simulink model "controller_dev_sg"  (R2018b)
settings: configuration reference "Physics" (kept outside this file)
model workspace (MAT data in the model file):
  m = 1000
undefined symbols (not defined in the file or in its folder): C, P_MLOC_NumberOfNoSendFrames, tS, TUMHealthStatus, TUMStateEstimationState, TUMVehicleState, x0_vehiclepose_stm
libraries: xpcrtudplib x13, simulink x12, canmsglib x12, etargetslib x10, speedgoatlib_IO614 x9, misc x4, xpcutilitieslib x1
(part 2 of 2)

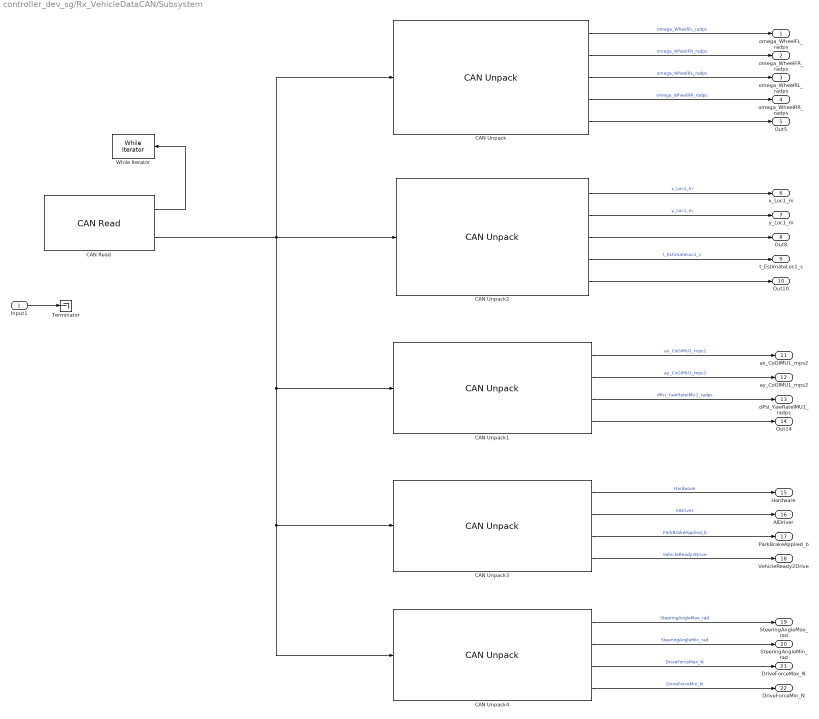
== system controller_dev_sg/Rx_VehicleDataCAN/Subsystem ==
  Input1 : Inport
  CAN Read : speedgoatlib_IO614/CAN/CAN Read  id=1  sampleTime=-1  portSelection=4  messageType=CAN  protl=IO614  ptIdx=3  isFDMod=0
      settings: SourceProductName=Simulink Real-Time: Speedgoat Library
  CAN Unpack : canmsglib/CAN Unpack  MsgList=(none)  MsgName=CAN Msg  MsgIDType=Standard (11-bit identifier)  MsgIdentifier=768  MsgLength=8  SignalInfo=omega_WheelFL_radps$0$15$1$1$1$0$0.1$0$-Inf$Inf$#omega_WheelFR_radps$15$15$1$1$1$0$0.1$0$-Inf$Inf$#omega_WheelRL_radps$30$15$1$1$1$0$0.1$0$-Inf$Inf$#omega_WheelRR_radps$45$15$1$1$1$0$0.1$0$-Inf$Inf$#valid_Wheelspeeds_b$60$4$1$1$1$0$1$0$-Inf$Inf$#  NSignals=5  IDPort=off  TimestampPort=off  ErrorPort=off  RemotePort=off  LengthPort=off  StatusPort=off  StartBits=str2num('[int32(0);int32(15);int32(30);int32(45);int32(60)]')  SignalSizes=str2num('[int32(15);int32(15);int32(15);int32(15);int32(4)]')  ByteOrders=str2num('[int32(1);int32(1);int32(1);int32(1);int32(1)]')  DataTypes=str2num('[int32(1);int32(1);int32(1);int32(1);int32(1)]')  MultiplexTypes=str2num('[int32(1);int32(1);int32(1);int32(1);int32(1)]')  MultiplexValues=str2num('[double(0);double(0);double(0);double(0);double(0)]')  Factors=str2num('[double(0.1);double(0.1);double(0.1);double(0.1);double(1)]')  Offsets=str2num('[double(0);double(0);double(0);double(0);double(0)]')  Minimums=str2num('[double(-Inf);double(-Inf);double(-Inf);double(-Inf);double(-Inf)]')  Maximums=str2num('[double(Inf);double(Inf);double(Inf);double(Inf);double(Inf)]')  ApplyMinMax=off
      settings: SourceProductName=Simulink Real-Time
  CAN Unpack1 : canmsglib/CAN Unpack  MsgList=(none)  MsgName=CAN Msg  MsgIDType=Standard (11-bit identifier)  MsgIdentifier=48  MsgLength=8  SignalInfo=ax_CoGIMU1_mps2$0$16$1$1$1$0$0.001$0$-Inf$Inf$#ay_CoGIMU1_mps2$16$16$1$1$1$0$0.001$0$-Inf$Inf$#dPsi_YawRateIMU1_radps$32$16$1$1$1$0$0.0001$0$-Inf$Inf$#valid_IMU1_b$48$16$1$1$1$0$1$0$-Inf$Inf$#  NSignals=4  IDPort=off  TimestampPort=off  ErrorPort=off  RemotePort=off  LengthPort=off  StatusPort=off  StartBits=str2num('[int32(0);int32(16);int32(32);int32(48)]')  SignalSizes=str2num('[int32(16);int32(16);int32(16);int32(16)]')  ByteOrders=str2num('[int32(1);int32(1);int32(1);int32(1)]')  DataTypes=str2num('[int32(1);int32(1);int32(1);int32(1)]')  MultiplexTypes=str2num('[int32(1);int32(1);int32(1);int32(1)]')  MultiplexValues=str2num('[double(0);double(0);double(0);double(0)]')  Factors=str2num('[double(0.001);double(0.001);double(0.0001);double(1)]')  Offsets=str2num('[double(0);double(0);double(0);double(0)]')  Minimums=str2num('[double(-Inf);double(-Inf);double(-Inf);double(-Inf)]')  Maximums=str2num('[double(Inf);double(Inf);double(Inf);double(Inf)]')  ApplyMinMax=off
      settings: SourceProductName=Simulink Real-Time
  CAN Unpack2 : canmsglib/CAN Unpack  MsgList=(none)  MsgName=CAN Msg  MsgIDType=Standard (11-bit identifier)  MsgIdentifier=192  MsgLength=8  SignalInfo=x_Loc1_m$0$15$1$1$1$0$0.05$0$-Inf$Inf$#y_Loc1_m$15$15$1$1$1$0$0.05$0$-Inf$Inf$#psi_YawAngleLoc1_rad$30$15$1$1$1$0$0.001$0$-Inf$Inf$#t_EstimateLoc1_s$45$15$1$1$1$0$0.001$0$-Inf$Inf$#valid_Loc1_b$60$4$1$1$1$0$1$0$-Inf$Inf$#  NSignals=5  IDPort=off  TimestampPort=off  ErrorPort=off  RemotePort=off  LengthPort=off  StatusPort=off  StartBits=str2num('[int32(0);int32(15);int32(30);int32(45);int32(60)]')  SignalSizes=str2num('[int32(15);int32(15);int32(15);int32(15);int32(4)]')  ByteOrders=str2num('[int32(1);int32(1);int32(1);int32(1);int32(1)]')  DataTypes=str2num('[int32(1);int32(1);int32(1);int32(1);int32(1)]')  MultiplexTypes=str2num('[int32(1);int32(1);int32(1);int32(1);int32(1)]')  MultiplexValues=str2num('[double(0);double(0);double(0);double(0);double(0)]')  Factors=str2num('[double(0.05);double(0.05);double(0.001);double(0.001);double(1)]')  Offsets=str2num('[double(0);double(0);double(0);double(0);double(0)]')  Minimums=str2num('[double(-Inf);double(-Inf);double(-Inf);double(-Inf);double(-Inf)]')  Maximums=str2num('[double(Inf);double(Inf);double(Inf);double(Inf);double(Inf)]')  ApplyMinMax=off
      settings: SourceProductName=Simulink Real-Time
  CAN Unpack3 : canmsglib/CAN Unpack  MsgList=(none)  MsgName=CAN Msg  MsgIDType=Standard (11-bit identifier)  MsgIdentifier=12  MsgLength=8  SignalInfo=Hardware$0$12$1$2$1$0$1$0$-Inf$Inf$#AIDriver$12$12$1$2$1$0$1$0$-Inf$Inf$#ParkBrakeApplied_b$24$12$1$1$1$0$1$0$-Inf$Inf$#VehicleReady2Drive$36$12$1$1$1$0$1$0$-Inf$Inf$#  NSignals=4  IDPort=off  TimestampPort=off  ErrorPort=off  RemotePort=off  LengthPort=off  StatusPort=off  StartBits=str2num('[int32(0);int32(12);int32(24);int32(36)]')  SignalSizes=str2num('[int32(12);int32(12);int32(12);int32(12)]')  ByteOrders=str2num('[int32(1);int32(1);int32(1);int32(1)]')  DataTypes=str2num('[int32(2);int32(2);int32(1);int32(1)]')  MultiplexTypes=str2num('[int32(1);int32(1);int32(1);int32(1)]')  MultiplexValues=str2num('[double(0);double(0);double(0);double(0)]')  Factors=str2num('[double(1);double(1);double(1);double(1)]')  Offsets=str2num('[double(0);double(0);double(0);double(0)]')  Minimums=str2num('[double(-Inf);double(-Inf);double(-Inf);double(-Inf)]')  Maximums=str2num('[double(Inf);double(Inf);double(Inf);double(Inf)]')  ApplyMinMax=off
      settings: SourceProductName=Simulink Real-Time
  CAN Unpack4 : canmsglib/CAN Unpack  MsgList=(none)  MsgName=CAN Msg  MsgIDType=Standard (11-bit identifier)  MsgIdentifier=170  MsgLength=8  SignalInfo=SteeringAngleMax_rad$0$16$1$1$1$0$0.001$0$-Inf$Inf$#SteeringAngleMin_rad$16$16$1$1$1$0$0.001$0$-Inf$Inf$#DriveForceMax_N$32$16$1$1$1$0$100$0$-Inf$Inf$#DriveForceMin_N$48$16$1$1$1$0$100$0$-Inf$Inf$#  NSignals=4  IDPort=off  TimestampPort=off  ErrorPort=off  RemotePort=off  LengthPort=off  StatusPort=off  StartBits=str2num('[int32(0);int32(16);int32(32);int32(48)]')  SignalSizes=str2num('[int32(16);int32(16);int32(16);int32(16)]')  ByteOrders=str2num('[int32(1);int32(1);int32(1);int32(1)]')  DataTypes=str2num('[int32(1);int32(1);int32(1);int32(1)]')  MultiplexTypes=str2num('[int32(1);int32(1);int32(1);int32(1)]')  MultiplexValues=str2num('[double(0);double(0);double(0);double(0)]')  Factors=str2num('[double(0.001);double(0.001);double(100);double(100)]')  Offsets=str2num('[double(0);double(0);double(0);double(0)]')  Minimums=str2num('[double(-Inf);double(-Inf);double(-Inf);double(-Inf)]')  Maximums=str2num('[double(Inf);double(Inf);double(Inf);double(Inf)]')  ApplyMinMax=off
      settings: SourceProductName=Simulink Real-Time
  Terminator : Terminator
  While Iterator : WhileIterator  MaxIters=501  WhileBlockType=do-while
  omega_WheelFL_radps : Outport
  omega_WheelFR_radps : Outport  Port=2
  omega_WheelRL_radps : Outport  Port=3
  omega_WheelRR_radps : Outport  Port=4
  Out5 : Outport  Port=5
  x_Loc1_m : Outport  Port=6
  y_Loc1_m : Outport  Port=7
  Out8 : Outport  Port=8
  t_EstimateLoc1_s : Outport  Port=9
  Out10 : Outport  Port=10
  ax_CoGIMU1_mps2 : Outport  Port=11
  ay_CoGIMU1_mps2 : Outport  Port=12
  dPsi_YawRateIMU1_radps : Outport  Port=13
  Out14 : Outport  Port=14
  Hardware : Outport  Port=15
  AIDriver : Outport  Port=16
  ParkBrakeApplied_b : Outport  Port=17
  VehicleReady2Drive : Outport  Port=18
  SteeringAngleMax_rad : Outport  Port=19
  SteeringAngleMin_rad : Outport  Port=20
  DriveForceMax_N : Outport  Port=21
  DriveForceMin_N : Outport  Port=22
  wires:
  CAN Read/2 -> CAN Unpack/1, CAN Unpack2/1, CAN Unpack1/1, CAN Unpack3/1, CAN Unpack4/1
  CAN Unpack/4 -> omega_WheelRR_radps/1  "omega_WheelRR_radps"
  CAN Unpack2/2 -> y_Loc1_m/1  "y_Loc1_m"
  CAN Unpack2/5 -> Out10/1
  Input1/1 -> Terminator/1
  CAN Unpack/5 -> Out5/1
  CAN Read/1 -> While Iterator/1
  CAN Unpack1/1 -> ax_CoGIMU1_mps2/1  "ax_CoGIMU1_mps2"
  CAN Unpack2/4 -> t_EstimateLoc1_s/1  "t_EstimateLoc1_s"
  CAN Unpack2/3 -> Out8/1
  CAN Unpack/1 -> omega_WheelFL_radps/1  "omega_WheelFL_radps"
  CAN Unpack4/3 -> DriveForceMax_N/1  "DriveForceMax_N"
  CAN Unpack/3 -> omega_WheelRL_radps/1  "omega_WheelRL_radps"
  CAN Unpack1/2 -> ay_CoGIMU1_mps2/1  "ay_CoGIMU1_mps2"
  CAN Unpack4/2 -> SteeringAngleMin_rad/1  "SteeringAngleMin_rad"
  CAN Unpack3/2 -> AIDriver/1  "AIDriver"
  CAN Unpack3/3 -> ParkBrakeApplied_b/1  "ParkBrakeApplied_b"
  CAN Unpack1/4 -> Out14/1
  CAN Unpack4/1 -> SteeringAngleMax_rad/1  "SteeringAngleMax_rad"
  CAN Unpack/2 -> omega_WheelFR_radps/1  "omega_WheelFR_radps"
  CAN Unpack2/1 -> x_Loc1_m/1  "x_Loc1_m"
  CAN Unpack3/4 -> VehicleReady2Drive/1  "VehicleReady2Drive"
  CAN Unpack3/1 -> Hardware/1  "Hardware"
  CAN Unpack1/3 -> dPsi_YawRateIMU1_radps/1  "dPsi_YawRateIMU1_radps"
  CAN Unpack4/4 -> DriveForceMin_N/1  "DriveForceMin_N"

== system controller_dev_sg/Tx_TPCommsControllerSide/BehaviorStatemachine ==
  TrajPlannerSend : Inport
  DebugData : Inport  Port=2  OutDataTypeStr=Bus: mvdc_vehicle_dynamics_control_debug  PortDimensions=1
  Bus Selector1 : BusSelector  OutputSignals=TUMVehicleState
  Bus Selector2 : BusSelector  OutputSignals=ErrorCode
  Byte Pack : etargetslib/Byte Pack  datatypes={'uint16', 'uint32', 'uint16'}  byteAlign=1
  Constant : Constant  Value=boolean(1)  SampleTime=-1
  Counter Free-Running : simulink/Sources/Counter Free-Running  NumBits=8  tsamp=-1
  Data Type Conversion : DataTypeConversion  OutDataTypeStr=uint16
  Data Type Conversion1 : DataTypeConversion  OutDataTypeStr=uint32
  Data Type Conversion2 : DataTypeConversion  OutDataTypeStr=uint16
  BSM_ActivateSend : Outport
  BSM_Package : Outport  Port=2
  wires:
  Counter Free-Running/1 -> Data Type Conversion2/1
  Data Type Conversion/1 -> Byte Pack/1
  Data Type Conversion2/1 -> Byte Pack/3
  Byte Pack/1 -> BSM_Package/1
  Constant/1 -> BSM_ActivateSend/1
  TrajPlannerSend/1 -> Bus Selector1/1
  Bus Selector1/1 -> Data Type Conversion/1  "<TUMVehicleState>"
  DebugData/1 -> Bus Selector2/1
  Bus Selector2/1 -> Data Type Conversion1/1  "<ErrorCode>"
  Data Type Conversion1/1 -> Byte Pack/2

== system controller_dev_sg/Tx_TPCommsControllerSide/SendToBehaviorStatemachine1 ==
  Data : Inport
  Enable : EnablePort
  "Send " : xpcrtudplib/UDP Send  ipAddressVal=10.0.1.0  localPort=-1  toAddress=255.255.255.255  toPort=BehaviorStatemachineSend_Port  sampleTime=-1
      settings: SourceProductName=Simulink Real-Time  SourceProductBaseCode=XP
  Width : Width
  wires:
  Width/1 -> "Send "/2
  Data/1 -> Width/1, "Send "/1

== system controller_dev_sg/Tx_TPCommsControllerSide/SendToTrajectoryGeneration1 ==
  Data : Inport
  Enable : EnablePort
  "Send " : xpcrtudplib/UDP Send  ipAddressVal=10.0.1.0  localPort=-1  toAddress=255.255.255.255  toPort=TrajectoryGenerationSend_Port  sampleTime=-1
      settings: SourceProductName=Simulink Real-Time  SourceProductBaseCode=XP
  Width : Width
  wires:
  Width/1 -> "Send "/2
  Data/1 -> Width/1, "Send "/1

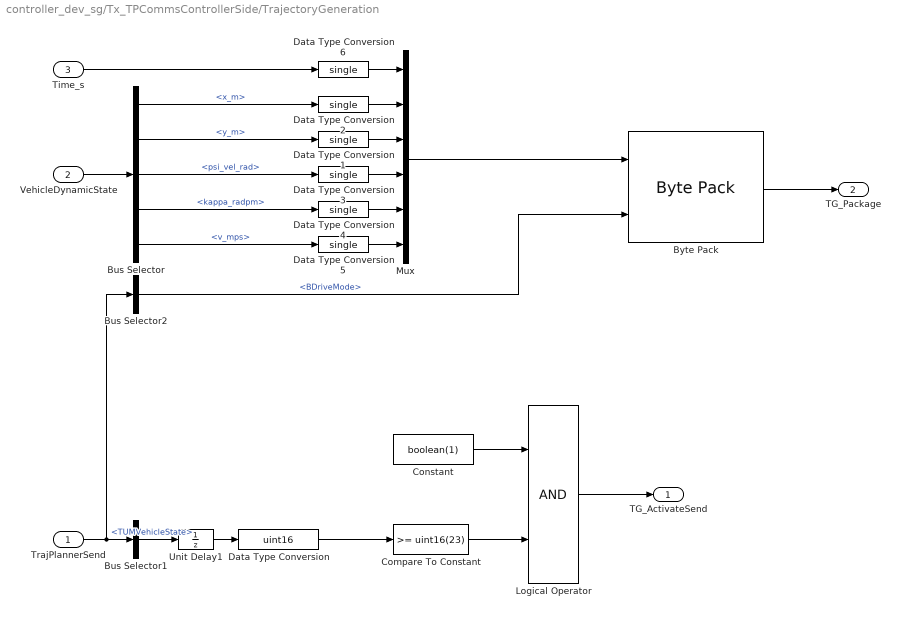
== system controller_dev_sg/Tx_TPCommsControllerSide/TrajectoryGeneration ==
  TrajPlannerSend : Inport
  VehicleDynamicState : Inport  Port=2
  Time_s : Inport  Port=3
  Bus Selector : BusSelector  OutputSignals=Pos.x_m,Pos.y_m,psi_vel_rad,kappa_radpm,v_mps
  Bus Selector1 : BusSelector  OutputSignals=TUMVehicleState
  Bus Selector2 : BusSelector  OutputSignals=BDriveMode
  Byte Pack : etargetslib/Byte Pack  datatypes={['single'], 'uint8'}  byteAlign=1
  Compare To Constant : simulink/Logic and Bit Operations/Compare To Constant  relop=>=  const=uint16(23)  OutDataTypeStr=boolean
  Constant : Constant  Value=boolean(1)  SampleTime=-1
  Data Type Conversion : DataTypeConversion  OutDataTypeStr=uint16
  Data Type Conversion{1..6} (6 alike) : DataTypeConversion  OutDataTypeStr=single
  Logical Operator : Logic  AllPortsSameDT=off  OutDataTypeStr=boolean
  Mux : Mux  Inputs=6
  Unit Delay1 : UnitDelay  InitialCondition=TUMVehicleState.OFF  SampleTime=tS
  TG_ActivateSend : Outport
  TG_Package : Outport  Port=2
  wires:
  Unit Delay1/1 -> Data Type Conversion/1
  Data Type Conversion/1 -> Compare To Constant/1
  Bus Selector/5 -> Data Type Conversion5/1  "<v_mps>"
  Data Type Conversion6/1 -> Mux/1
  Data Type Conversion4/1 -> Mux/5
  Data Type Conversion5/1 -> Mux/6
  Data Type Conversion1/1 -> Mux/3
  Data Type Conversion2/1 -> Mux/2
  Data Type Conversion3/1 -> Mux/4
  Time_s/1 -> Data Type Conversion6/1
  VehicleDynamicState/1 -> Bus Selector/1
  Mux/1 -> Byte Pack/1
  Bus Selector/4 -> Data Type Conversion4/1  "<kappa_radpm>"
  Byte Pack/1 -> TG_Package/1
  Bus Selector/1 -> Data Type Conversion2/1  "<x_m>"
  Bus Selector/2 -> Data Type Conversion1/1  "<y_m>"
  Bus Selector/3 -> Data Type Conversion3/1  "<psi_vel_rad>"
  Compare To Constant/1 -> Logical Operator/2
  Logical Operator/1 -> TG_ActivateSend/1
  Constant/1 -> Logical Operator/1
  TrajPlannerSend/1 -> Bus Selector2/1, Bus Selector1/1
  Bus Selector1/1 -> Unit Delay1/1  "<TUMVehicleState>"
  Bus Selector2/1 -> Byte Pack/2  "<BDriveMode>"

== system controller_dev_sg/Tx_TPCommsTPSide/BSM_Package ==
  TrajPlannerSend : Inport
  Bus Selector : BusSelector  OutputSignals=Strategy_Status
  Byte Pack : etargetslib/Byte Pack  datatypes={'uint16', 'uint16', 'uint32'}  byteAlign=1
  Constant : Constant  Value=0  SampleTime=-1
  Counter Free-Running : simulink/Sources/Counter Free-Running  NumBits=8  tsamp=-1
  Data Type Conversion : DataTypeConversion  OutDataTypeStr=uint16
  Data Type Conversion1 : DataTypeConversion  OutDataTypeStr=uint32
  Data Type Conversion2 : DataTypeConversion  OutDataTypeStr=uint16
  ResettableCounter : Subsystem
  BSM_ActivateSend : Outport
  BSM_Package : Outport  Port=2
  wires:
  Byte Pack/1 -> BSM_Package/1
  ResettableCounter/1(BSMActivateSend) -> BSM_ActivateSend/1
  TrajPlannerSend/1 -> Bus Selector/1
  Bus Selector/1 -> Data Type Conversion/1  "<Strategy_Status>"
  Data Type Conversion/1 -> Byte Pack/1
  Data Type Conversion1/1 -> Byte Pack/3
  Constant/1 -> Data Type Conversion1/1
  Counter Free-Running/1 -> Data Type Conversion2/1
  Data Type Conversion2/1 -> Byte Pack/2

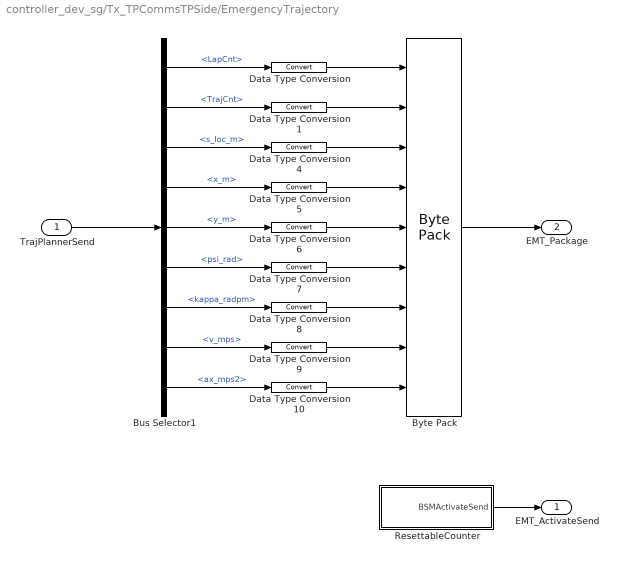
== system controller_dev_sg/Tx_TPCommsTPSide/EmergencyTrajectory ==
  TrajPlannerSend : Inport
  Bus Selector1 : BusSelector  OutputSignals=EmergencyTrajectory.LapCnt,EmergencyTrajectory.TrajCnt,EmergencyTrajectory.s_loc_m,EmergencyTrajectory.x_m,EmergencyTrajectory.y_m,EmergencyTrajectory.psi_rad,EmergencyTrajectory.kappa_radpm,EmergencyTrajectory.v_mps,EmergencyTrajectory.ax_mps2
  Byte Pack : etargetslib/Byte Pack  datatypes={'uint32', 'uint32', ['single'], ['single'], ['single'], ['single'], ['single'], ['single'], ['single']}  byteAlign=1
  Data Type Conversion{,1,4..10} (9 alike) : DataTypeConversion
  ResettableCounter : Subsystem
  EMT_ActivateSend : Outport
  EMT_Package : Outport  Port=2
  wires:
  Byte Pack/1 -> EMT_Package/1
  ResettableCounter/1(BSMActivateSend) -> EMT_ActivateSend/1
  TrajPlannerSend/1 -> Bus Selector1/1
  Bus Selector1/1 -> Data Type Conversion/1  "<LapCnt>"
  Bus Selector1/2 -> Data Type Conversion1/1  "<TrajCnt>"
  Bus Selector1/3 -> Data Type Conversion4/1  "<s_loc_m>"
  Bus Selector1/4 -> Data Type Conversion5/1  "<x_m>"
  Bus Selector1/5 -> Data Type Conversion6/1  "<y_m>"
  Bus Selector1/6 -> Data Type Conversion7/1  "<psi_rad>"
  Bus Selector1/7 -> Data Type Conversion8/1  "<kappa_radpm>"
  Bus Selector1/8 -> Data Type Conversion9/1  "<v_mps>"
  Bus Selector1/9 -> Data Type Conversion10/1  "<ax_mps2>"
  Data Type Conversion/1 -> Byte Pack/1
  Data Type Conversion1/1 -> Byte Pack/2
  Data Type Conversion10/1 -> Byte Pack/9
  Data Type Conversion9/1 -> Byte Pack/8
  Data Type Conversion8/1 -> Byte Pack/7
  Data Type Conversion7/1 -> Byte Pack/6
  Data Type Conversion6/1 -> Byte Pack/5
  Data Type Conversion5/1 -> Byte Pack/4
  Data Type Conversion4/1 -> Byte Pack/3

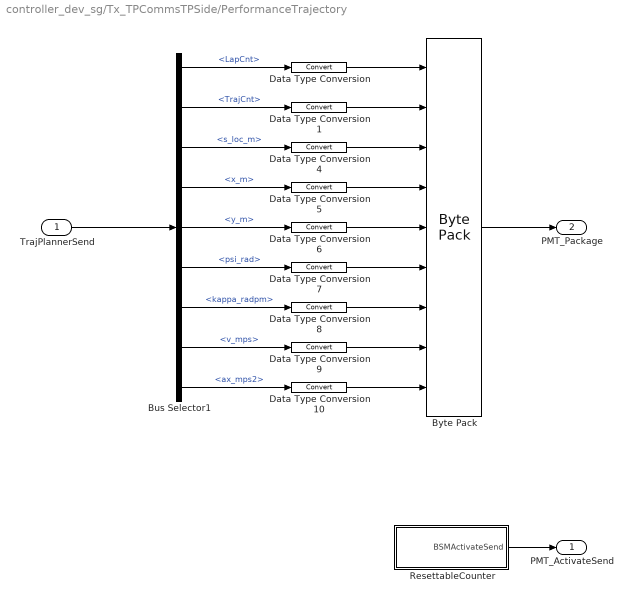
== system controller_dev_sg/Tx_TPCommsTPSide/PerformanceTrajectory ==
  TrajPlannerSend : Inport
  Bus Selector1 : BusSelector  OutputSignals=PerformanceTrajectory.LapCnt,PerformanceTrajectory.TrajCnt,PerformanceTrajectory.s_loc_m,PerformanceTrajectory.x_m,PerformanceTrajectory.y_m,PerformanceTrajectory.psi_rad,PerformanceTrajectory.kappa_radpm,PerformanceTrajectory.v_mps,PerformanceTrajectory.ax_mps2
  Byte Pack : etargetslib/Byte Pack  datatypes={'uint32', 'uint32', ['single'], ['single'], ['single'], ['single'], ['single'], ['single'], ['single']}  byteAlign=1
  Data Type Conversion{,1,4..10} (9 alike) : DataTypeConversion
  ResettableCounter : Subsystem
  PMT_ActivateSend : Outport
  PMT_Package : Outport  Port=2
  wires:
  ResettableCounter/1(BSMActivateSend) -> PMT_ActivateSend/1
  TrajPlannerSend/1 -> Bus Selector1/1
  Data Type Conversion1/1 -> Byte Pack/2
  Bus Selector1/9 -> Data Type Conversion10/1  "<ax_mps2>"
  Bus Selector1/4 -> Data Type Conversion5/1  "<x_m>"
  Bus Selector1/2 -> Data Type Conversion1/1  "<TrajCnt>"
  Bus Selector1/1 -> Data Type Conversion/1  "<LapCnt>"
  Bus Selector1/7 -> Data Type Conversion8/1  "<kappa_radpm>"
  Bus Selector1/6 -> Data Type Conversion7/1  "<psi_rad>"
  Bus Selector1/5 -> Data Type Conversion6/1  "<y_m>"
  Data Type Conversion/1 -> Byte Pack/1
  Bus Selector1/8 -> Data Type Conversion9/1  "<v_mps>"
  Data Type Conversion10/1 -> Byte Pack/9
  Bus Selector1/3 -> Data Type Conversion4/1  "<s_loc_m>"
  Data Type Conversion5/1 -> Byte Pack/4
  Data Type Conversion6/1 -> Byte Pack/5
  Data Type Conversion7/1 -> Byte Pack/6
  Data Type Conversion4/1 -> Byte Pack/3
  Byte Pack/1 -> PMT_Package/1
  Data Type Conversion8/1 -> Byte Pack/7
  Data Type Conversion9/1 -> Byte Pack/8

== system controller_dev_sg/Tx_TPCommsTPSide/SendBehaviorStateMachine ==
  Data : Inport
  Enable : EnablePort
  "Send " : xpcrtudplib/UDP Send  ipAddressVal=10.0.2.0  localPort=-1  toAddress=255.255.255.255  toPort=BehaviorStatemachineSend_Port  sampleTime=-1
      settings: SourceProductName=Simulink Real-Time  SourceProductBaseCode=XP
  Width : Width
  wires:
  Width/1 -> "Send "/2
  Data/1 -> Width/1, "Send "/1

== system controller_dev_sg/Tx_TPCommsTPSide/SendEmergencyTrajectory ==
  Data : Inport
  Enable : EnablePort
  "Send " : xpcrtudplib/UDP Send  ipAddressVal=10.0.2.0  localPort=-1  toAddress=255.255.255.255  toPort=EmergencyPathRcv_Port  sampleTime=-1
      settings: SourceProductName=Simulink Real-Time  SourceProductBaseCode=XP
  Width : Width
  wires:
  Width/1 -> "Send "/2
  Data/1 -> Width/1, "Send "/1

== system controller_dev_sg/Tx_TPCommsTPSide/SendPerformanceTrajectory ==
  Data : Inport
  Enable : EnablePort
  "Send " : xpcrtudplib/UDP Send  ipAddressVal=10.0.2.0  localPort=-1  toAddress=255.255.255.255  toPort=PerformanceTrajectoryRcv_Port  sampleTime=-1
      settings: SourceProductName=Simulink Real-Time  SourceProductBaseCode=XP
  Width : Width
  wires:
  Width/1 -> "Send "/2
  Data/1 -> Width/1, "Send "/1

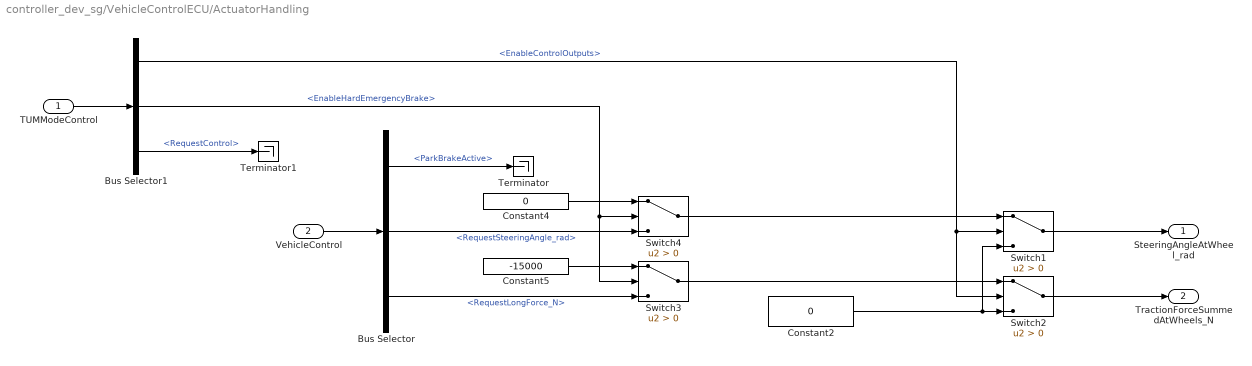
== system controller_dev_sg/VehicleControlECU/ActuatorHandling ==
  TUMModeControl : Inport  OutDataTypeStr=Bus: TUMModeControl
  VehicleControl : Inport  Port=2  OutDataTypeStr=Bus: VehicleControl
  Bus Selector : BusSelector  OutputSignals=ParkBrakeActive,RequestSteeringAngle_rad,RequestLongForce_N
  Bus Selector1 : BusSelector  OutputSignals=EnableControlOutputs,EnableHardEmergencyBrake,RequestControl
  Constant2 : Constant  Value=0
  Constant4 : Constant  Value=0
  Constant5 : Constant  Value=-15000
  Switch{1..4} (4 alike) : Switch  Criteria=u2 > Threshold
  Terminator : Terminator
  Terminator1 : Terminator
  SteeringAngleAtWheel_rad : Outport
  TractionForceSummedAtWheels_N : Outport  Port=2
  wires:
  Bus Selector1/1 -> Switch2/2, Switch1/2  "<EnableControlOutputs>"
  TUMModeControl/1 -> Bus Selector1/1
  Bus Selector/3 -> Switch3/3  "<RequestLongForce_N>"
  Constant2/1 -> Switch1/3, Switch2/3
  VehicleControl/1 -> Bus Selector/1
  Bus Selector/2 -> Switch4/3  "<RequestSteeringAngle_rad>"
  Constant4/1 -> Switch4/1
  Constant5/1 -> Switch3/1
  Bus Selector1/2 -> Switch3/2, Switch4/2  "<EnableHardEmergencyBrake>"
  Bus Selector/1 -> Terminator/1  "<ParkBrakeActive>"
  Bus Selector1/3 -> Terminator1/1  "<RequestControl>"
  Switch4/1 -> Switch1/1
  Switch3/1 -> Switch2/1
  Switch1/1 -> SteeringAngleAtWheel_rad/1
  Switch2/1 -> TractionForceSummedAtWheels_N/1

== system controller_dev_sg/Tx_TPCommsTPSide/BSM_Package/ResettableCounter ==
  Compare To Constant : simulink/Logic and Bit Operations/Compare To Constant  relop=>=  const=5  OutDataTypeStr=boolean
  Constant : Constant
  Constant1 : Constant  Value=0
  Sum : Sum  Inputs=|++
  Switch : Switch  Criteria=u2 ~= 0  Threshold=P_MLOC_NumberOfNoSendFrames
  Unit Delay : UnitDelay  SampleTime=-1
  BSMActivateSend : Outport
  wires:
  Unit Delay/1 -> Compare To Constant/1, Sum/2
  Compare To Constant/1 -> BSMActivateSend/1, Switch/2
  Switch/1 -> Unit Delay/1
  Constant/1 -> Sum/1
  Constant1/1 -> Switch/1
  Sum/1 -> Switch/3

== system controller_dev_sg/Tx_TPCommsTPSide/EmergencyTrajectory/ResettableCounter ==
  Compare To Constant : simulink/Logic and Bit Operations/Compare To Constant  relop=>=  const=5  OutDataTypeStr=boolean
  Constant : Constant  SampleTime=-1
  Constant1 : Constant  Value=0  SampleTime=-1
  Sum : Sum  Inputs=|++
  Switch : Switch  Criteria=u2 ~= 0  Threshold=P_MLOC_NumberOfNoSendFrames
  Unit Delay : UnitDelay  SampleTime=-1
  BSMActivateSend : Outport
  wires:
  Unit Delay/1 -> Compare To Constant/1, Sum/2
  Compare To Constant/1 -> BSMActivateSend/1, Switch/2
  Switch/1 -> Unit Delay/1
  Constant/1 -> Sum/1
  Constant1/1 -> Switch/1
  Sum/1 -> Switch/3

== system controller_dev_sg/Tx_TPCommsTPSide/PerformanceTrajectory/ResettableCounter ==
  Compare To Constant : simulink/Logic and Bit Operations/Compare To Constant  relop=>=  const=5  OutDataTypeStr=boolean
  Constant : Constant  SampleTime=-1
  Constant1 : Constant  Value=0  SampleTime=-1
  Sum : Sum  Inputs=|++
  Switch : Switch  Criteria=u2 ~= 0  Threshold=P_MLOC_NumberOfNoSendFrames
  Unit Delay : UnitDelay  SampleTime=-1
  BSMActivateSend : Outport
  wires:
  Unit Delay/1 -> Compare To Constant/1, Sum/2
  Compare To Constant/1 -> BSMActivateSend/1, Switch/2
  Switch/1 -> Unit Delay/1
  Constant/1 -> Sum/1
  Constant1/1 -> Switch/1
  Sum/1 -> Switch/3
